simulink model "Orbit_prop_279C_v1"  (R2018b)
settings: Solver=ode113  StartTime=0.0  StopTime=3600*24*176.9228*omega  FixedStep=2  MaxStep=25 * omega  RelTol=1e-10  AbsTol=1e-12
values from neighbouring files (symbols this model uses):
  C = eye(3)    [PSet3_eml.m]    (also in Pset3_Orbit_prop.m = [.892539 .157379 -.422618 -.275451 0.932257 -.234570 .357073; Pset3_Orbit_prop_dim.m; gif_test.m = [.892539 .157379 -.422618; -.275451 0.932257 -.234570; .3570)
  I_vec = [sc.Ip(1,1); sc.Ip(2,2); sc.Ip(3,3)]    [Compare_run.m]    (also in PSet2_eml.m; PSet3_eml.m; Pset3_Orbit_prop.m; Pset3_Orbit_prop_dim.m)
  mu1 = 328900.56^-1    (= 3.04043264627e-06)    [Compare_run.m]    (also in PSet1.m; Pset3_Orbit_prop.m; Pset3_Orbit_prop_dim.m; Pset_4_TD.m)
  r0 = [.98900883730044109; 0; 0.000802140914099732]*dis.sun    [Compare_run.m]    (also in Pset3_Orbit_prop.m = [.98900883730044109; 0; 0.000802140914099732]; Pset3_Orbit_prop_dim.m; Pset_4_TD.m; Sim_Run_File.m)
  v0 = [0; 0.010697471710460349-2.895683e-3; 0] * dis.sun * omega    [Compare_run.m]    (also in Pset3_Orbit_prop.m = [0; 0.010697471710460349-3.24371e-3; 0]; Pset3_Orbit_prop_dim.m; Pset_4_TD.m; Sim_Run_File.m)
  w0 = [1; 1; 1]*pi/180    [Compare_run.m]    (also in Pset3_Orbit_prop.m = [.001; .001; 5] * pi()/180; Pset3_Orbit_prop_dim.m = [2; 1; 2.5] * pi()/180; Pset_4_TD.m = [omega/100 ; omega;  omega/100]; Sim_Run_File.m = [0.2; 2; 0.2]*pi/180)
settings Model: Creator=ayotundedemuren  LastModifiedBy=Ethan
settings SolverCC: AutoScaleAbsTol=off

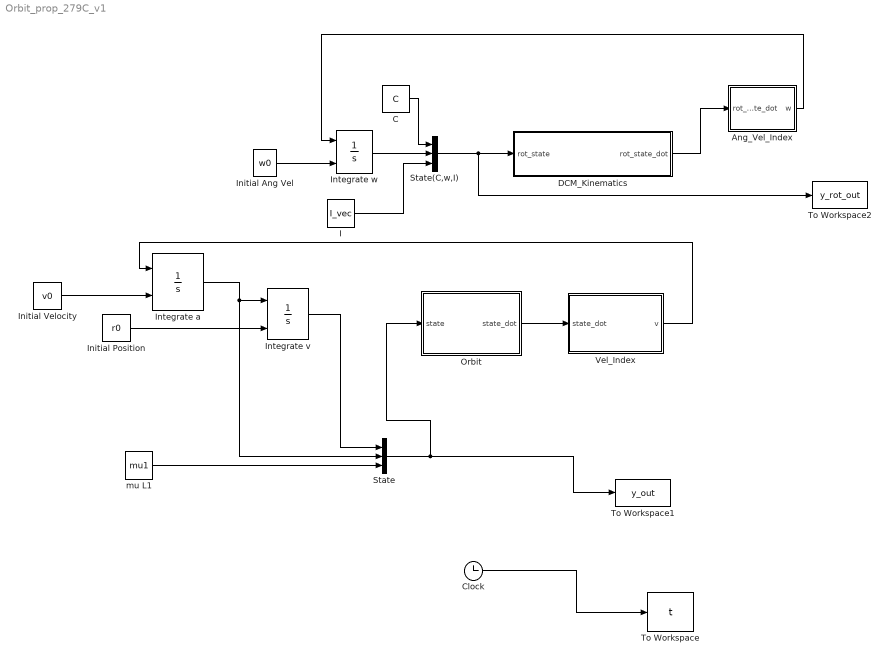
== system Orbit_prop_279C_v1 ==
  Ang_Vel_Index : MATLAB Function  TreatAsAtomicUnit=on
  C : Constant  Value=C
  Clock : Clock
  DCM_Kinematics : MATLAB Function  TreatAsAtomicUnit=on
  I : Constant  Value=I_vec
  Initial Ang Vel : Constant  Value=w0
  Initial Position : Constant  Value=r0
  Initial Velocity : Constant  Value=v0
  Integrate a : Integrator  InitialConditionSource=external  AbsoluteTolerance=1e-6
  Integrate v : Integrator  InitialConditionSource=external  AbsoluteTolerance=1e-6
  Integrate w : Integrator  InitialConditionSource=external
  Orbit : MATLAB Function  TreatAsAtomicUnit=on
  "State " : Concatenate  NumInputs=3
  State(C,w,I) : Concatenate  NumInputs=3
  To Workspace : ToWorkspace  VariableName=t  SampleTime=-1
      settings: Save2DSignal=2-D array (concatenate along first dimension)
  To Workspace1 : ToWorkspace  VariableName=y_out  SampleTime=-1
  To Workspace2 : ToWorkspace  VariableName=y_rot_out  SampleTime=-1
  Vel_Index : MATLAB Function  TreatAsAtomicUnit=on
  mu L1 : Constant  Value=mu1
  wires:
  Initial Velocity/1 -> Integrate a/2
  Initial Position/1 -> Integrate v/2
  Integrate v/1 -> "State "/1
  Vel_Index/1(v) -> Integrate a/1
  "State "/1 -> Orbit/1(state), To Workspace1/1
  Integrate a/1 -> Integrate v/1, "State "/2
  mu L1/1 -> "State "/3
  Orbit/1(state_dot) -> Vel_Index/1(state_dot)
  Initial Ang Vel/1 -> Integrate w/2
  State(C,w,I)/1 -> To Workspace2/1, DCM_Kinematics/1(rot_state)
  Integrate w/1 -> State(C,w,I)/2
  C/1 -> State(C,w,I)/1
  I/1 -> State(C,w,I)/3
  DCM_Kinematics/1(rot_state_dot) -> Ang_Vel_Index/1(rot_state_dot)
  Ang_Vel_Index/1(w) -> Integrate w/1
  Clock/1 -> To Workspace/1

== matlab function Orbit_prop_279C_v1/Vel_Index ==
  data: state_dot input; v output
function v = fcn(state_dot)

v = state_dot(4:6);

end

== matlab function Orbit_prop_279C_v1/Orbit ==
  data: state input; state_dot output
function state_dot = fcn(state)

state_dot = zeros(7,1);
x = state(1);
y = state(2);
z = state(3);
xdot = state(4);
ydot = state(5);
zdot = state(6);

mu = state(7);

rho1 = sqrt((x + mu)^2 + y^2 + z^2);
rho2 = sqrt((x - (1-mu))^2 + y^2 + z^2);

state_dot(1) = xdot;
state_dot(2) = ydot;
state_dot(3) = zdot;

state_dot(4) = x + 2*ydot - (1 - mu)*(x + mu)/rho1^3 - ...
    mu*(x - (1 - mu))/rho2^3;
state_dot(5) = y - 2*xdot - (1 - mu)*(y)/rho1^3 - ...
    mu*(y)/rho2^3;
state_dot(6) = -(1 - mu)*z/rho1^3 - mu*z/rho2^3;
for ii = 4:6
    if abs(state_dot(ii)) < 1e-15
        state_dot(ii) = 0;
    end
end
end

== matlab function Orbit_prop_279C_v1/DCM_Kinematics ==
  data: rot_state input; rot_state_dot output
function rot_state_dot  = DCM_kin(rot_state)
% state = [C(:) w1 w2 w3 I1 I2 I3]

rot_state_dot = zeros(length(rot_state),1);
wx = rot_state(10);
wy = rot_state(11);
wz = rot_state(12);
Ix = rot_state(13);
Iy = rot_state(14);
Iz = rot_state(15);
%% Kinematic Equations
Omega = [0 -wz wy; wz 0 -wx; -wy wx 0];
A = [rot_state(1) rot_state(4) rot_state(7); rot_state(2) rot_state(5) rot_state(8); rot_state(3)...
    rot_state(6) rot_state(9)];
rot_state_dot(1:9) = -Omega * A;

%% Euler Equations
rot_state_dot(10) = -wy*wz * (Iz - Iy)/Ix;
rot_state_dot(11) = -wx*wz * (Ix - Iz)/Iy;
rot_state_dot(12) = -wx*wy * (Iy - Ix)/Iz;

end

== matlab function Orbit_prop_279C_v1/Ang_Vel_Index ==
  data: rot_state_dot input; w output
function w = fcn(rot_state_dot)

w = rot_state_dot(10:12);

end
